simulink model "equal_area_criterion"  (R2014a)
settings: Solver=ode23t  StartTime=0.0  StopTime=1  RelTol=1e-3
settings Model: Creator=Divya M  LastModifiedBy=Divya M

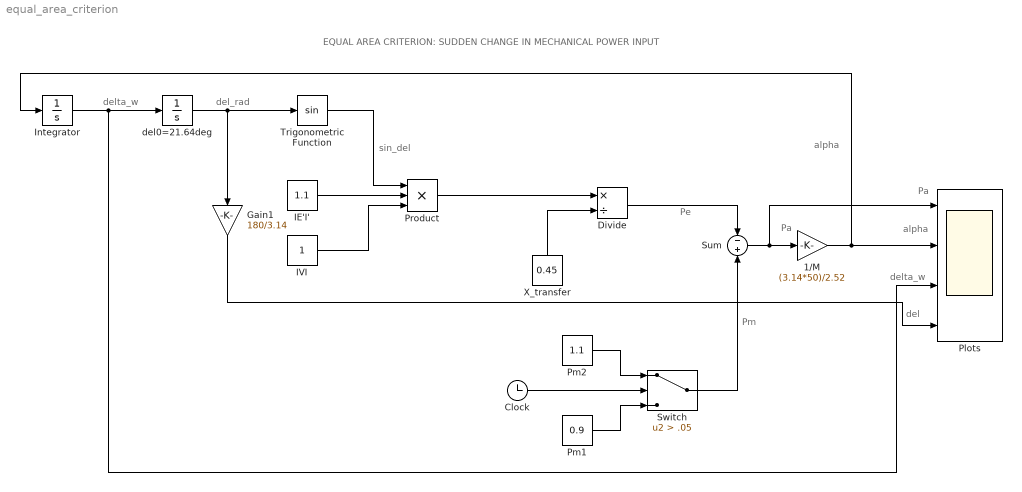
== system equal_area_criterion ==
  note: Pm
  note: del
  note: delta_w
  note: alpha
  note: Pa
  note: alpha
  note: Pa
  note: Pe
  note: sin_del
  note: del_rad
  note: delta_w
  note: EQUAL AREA CRITERION: SUDDEN CHANGE IN MECHANICAL POWER INPUT
  1/M : Gain  Gain=(3.14*50)/2.52
  Clock : Clock
  Divide : Product  Inputs=*/
  Gain1 : Gain  Gain=180/3.14
  IE'I' : Constant  Value=1.1
  IVI : Constant
  Integrator : Integrator
  Plots : Scope  NumInputPorts=4
      settings: YMin=-0.3~-1000~-10~20  YMax=0.3~1000~10~35
  Pm1 : Constant  Value=0.9
  Pm2 : Constant  Value=1.1
  Product : Product  Inputs=3
  Sum : Sum  Inputs=-+
  Switch : Switch  Criteria=u2 > Threshold  Threshold=.05
  Trigonometric Function : Trigonometry
  X_transfer : Constant  Value=0.45
  del0=21.64deg : Integrator  InitialCondition=(21.64*3.14)/180
  wires:
  Integrator/1 -> Plots/3, del0=21.64deg/1
  del0=21.64deg/1 -> Gain1/1, Trigonometric Function/1
  Trigonometric Function/1 -> Product/1
  IE'I'/1 -> Product/2
  IVI/1 -> Product/3
  Product/1 -> Divide/1
  Pm2/1 -> Switch/1
  Clock/1 -> Switch/2
  Pm1/1 -> Switch/3
  1/M/1 -> Plots/2, Integrator/1
  Divide/1 -> Sum/1
  X_transfer/1 -> Divide/2
  Switch/1 -> Sum/2
  Sum/1 -> Plots/1, 1/M/1
  Gain1/1 -> Plots/4
